simulink model "projet_simulink"  (R2021a)
settings: Solver=VariableStepAuto  StartTime=0.0  StopTime=100  RelTol=1e-3
values from neighbouring files (symbols this model uses):
  A = [0 1 0 ... (first row only)    [script_projet.m]
  B = [0;0;1]    [script_projet.m]
  C = [6.563 0 0 ]    [script_projet.m]
  k = place(A,B,p)    [script_projet.m]
  S = [ 1 X(2) X(3)]    [script_projet.m]
  T = 46.65*O    [script_projet.m]
libraries: eeAlternativeControllers x1
settings Model: Creator=Ghanem  LastModifiedBy=Ghanem

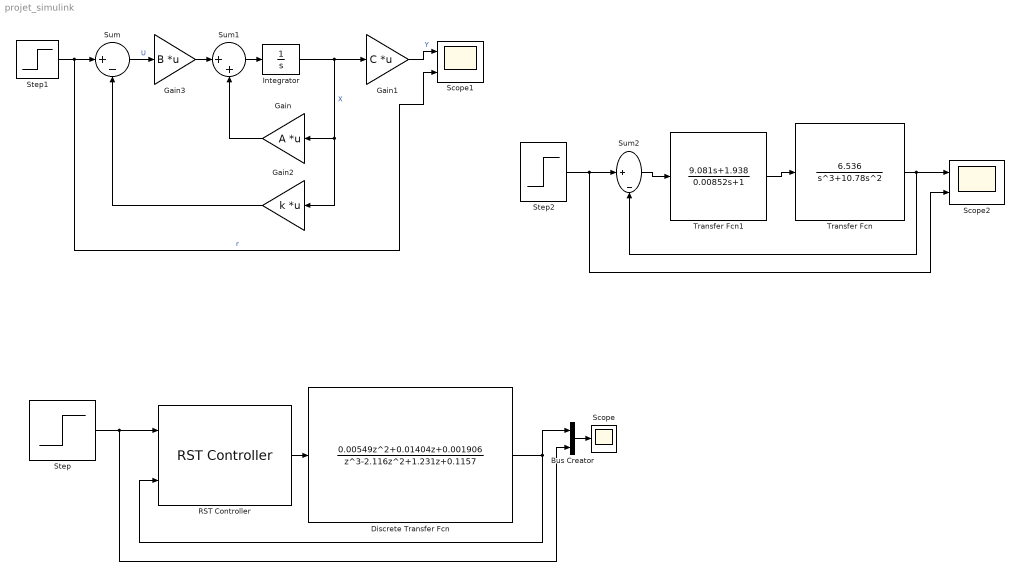
== system projet_simulink ==
  Bus Creator : BusCreator  Inputs=2
  Discrete Transfer Fcn : DiscreteTransferFcn  Numerator=[0.00549 0.01404 0.001906]  Denominator=[1 -2.116 1.231 0.1157]
  Gain : Gain  Gain=A  Multiplication=Matrix(K*u)
  Gain1 : Gain  Gain=C  Multiplication=Matrix(K*u) (u vector)
  Gain2 : Gain  Gain=k  Multiplication=Matrix(K*u) (u vector)
  Gain3 : Gain  Gain=B  Multiplication=Matrix(K*u) (u vector)
  Integrator : Integrator
  RST Controller : eeAlternativeControllers/RST Controller  CtrlParam=Controller polynomials  R=S  S=R  T=T  B=1  A=[1 0.5]  N=5  lam=0.5  d=2  Ts=-1
      settings: SourceProductBaseCode=PS
  Scope : Scope
  Scope1 : Scope  NumInputPorts=2
  Scope2 : Scope  NumInputPorts=2
  Step : Step  Before=1  SampleTime=0
  Step1 : Step  Time=0  SampleTime=0
  Step2 : Step  Time=0  SampleTime=0
  Sum : Sum  Inputs=|+-
  Sum1 : Sum  Inputs=|++
  Sum2 : Sum  Inputs=|+-
  Transfer Fcn : TransferFcn  Numerator=[6.536]  Denominator=[1 10.78 0 0]
  Transfer Fcn1 : TransferFcn  Numerator=[9.081 1.938]  Denominator=[0.00852 1]
  wires:
  Gain3/1 -> Sum1/1
  Gain/1 -> Sum1/2
  Gain2/1 -> Sum/2
  Integrator/1 -> Gain2/1, Gain/1, Gain1/1  "X"
  Sum1/1 -> Integrator/1
  Sum/1 -> Gain3/1  "U"
  Gain1/1 -> Scope1/1  "Y"
  Step1/1 -> Scope1/2, Sum/1  "r"
  Discrete Transfer Fcn/1 -> Bus Creator/1, RST Controller/2
  Bus Creator/1 -> Scope/1
  RST Controller/1 -> Discrete Transfer Fcn/1
  Step/1 -> Bus Creator/2, RST Controller/1
  Sum2/1 -> Transfer Fcn1/1
  Transfer Fcn1/1 -> Transfer Fcn/1
  Transfer Fcn/1 -> Scope2/1, Sum2/2
  Step2/1 -> Scope2/2, Sum2/1
